simulink model "initial_model2a"  (R2017b)
settings: Solver=ode4  StartTime=0.0  StopTime=time_final  FixedStep=time_step  RelTol=1e-3  AbsTol=1e-6
values from neighbouring files (symbols this model uses):
  A_frontal = 2.8    [tesla_sim_data2.m]    (also in tesla_sim_data2a.m)
  ap00 = -69.58    [tesla_sim_data2.m]    (also in tesla_sim_data2a.m)
  ap01 = 11.22    [tesla_sim_data2.m]    (also in tesla_sim_data2a.m)
  ap02 = -0.1665    [tesla_sim_data2.m]    (also in tesla_sim_data2a.m)
  ap03 = 0.0006218    [tesla_sim_data2.m]    (also in tesla_sim_data2a.m)
  ap10 = 0.5123    [tesla_sim_data2.m]    (also in tesla_sim_data2a.m)
  ap11 = 0.009736    [tesla_sim_data2.m]    (also in tesla_sim_data2a.m)
  ap12 = 0.0003316    [tesla_sim_data2.m]    (also in tesla_sim_data2a.m)
  ap20 = -0.0007943    [tesla_sim_data2.m]    (also in tesla_sim_data2a.m)
  ap21 = -4.587e-07    [tesla_sim_data2.m]    (also in tesla_sim_data2a.m)
  ap30 = 3.794e-07    [tesla_sim_data2.m]    (also in tesla_sim_data2a.m)
  C_d = 0.24    [tesla_sim_data2.m]    (also in tesla_sim_data2a.m)
  enable_stop = 1    [tesla_sim_data2.m]    (also in tesla_sim_data2a.m)
  ess_cap_scale = 1    [tesla_sim_data2.m]    (also in tesla_sim_data2a.m)
  ess_fixtemp = 25    [tesla_sim_data2.m]    (also in tesla_sim_data2a.m)
  ess_max_ah_cap = ess_max_kwhr_cap*1000/350*[1 1]    [tesla_sim_data2.m]    (also in tesla_sim_data2a.m)
  ess_max_volts = 9    [tesla_sim_data2.m]    (also in tesla_sim_data2a.m)
  ess_min_volts = 6    [tesla_sim_data2.m]    (also in tesla_sim_data2a.m)
  ess_module_num = 40    [tesla_sim_data2.m]    (also in tesla_sim_data2a.m)
  ess_r_chg = [ ... (first row only)    [tesla_sim_data2.m]    (also in tesla_sim_data2a.m)
  ess_r_dis = [ ... (first row only)    [tesla_sim_data2.m]    (also in tesla_sim_data2a.m)
  ess_res_scale_coef = [1 0 1 0]    [tesla_sim_data2.m]    (also in tesla_sim_data2a.m)
  ess_res_scale_fun = inline('(x(1)*ess_module_num+x(2))/(x(3)*ess_cap_scale+x(4))','x','ess_module_num','ess_cap_scale')    [tesla_sim_data2.m]    (also in tesla_sim_data2a.m)
  ess_soc = [0 0.1 0.2 0.3 0.4 0.5 0.6 0.7 0.8 0.9 1]    [tesla_sim_data2.m]    (also in tesla_sim_data2a.m)
  ess_tmp = [0 25]    [tesla_sim_data2.m]    (also in tesla_sim_data2a.m)
  ess_voc = [ ... (first row only)    [tesla_sim_data2.m]    (also in tesla_sim_data2a.m)
  f_rolling = 0.018    [tesla_sim_data2.m]    (also in tesla_sim_data2a.m)
  FR = 9.73    [tesla_sim_data2.m]    (also in tesla_sim_data2a.m)
  g_gravity = 9.81    [tesla_sim_data2.m]    (also in tesla_sim_data2a.m)
  m_map_spd = [0	100	250	500	1000	1500	2000	2500	3000	4000	4500	5500	6000	7000	8000	9000	10000]*(2*pi)/60    [tesla_sim_data2.m]    (also in tesla_sim_data2a.m)
  m_max_trq_IM = min(m_peak_trq_IM, m_peak_pwr*1000./m_map_spd)    [tesla_sim_data2.m]    (also in tesla_sim_data2a.m)
  m_max_trq_SR = min(m_peak_trq_SR, m_peak_pwr*1000./m_map_spd)    [tesla_sim_data2.m]    (also in tesla_sim_data2a.m)
  m_min_volts = 200    [tesla_sim_data2.m]    (also in tesla_sim_data2a.m)
  m_peak_pwr = 310    [tesla_sim_data2.m]    (also in tesla_sim_data2a.m)
  M_total = (4650+300)/2.2046    (= 2245.3052708)    [tesla_sim_data2.m]    (also in tesla_sim_data2a.m)
  mtr_speed_rad = linspace(0,6000*2*pi/60,d)    [tesla_sim_data2.m]    (also in tesla_sim_data2a.m = linspace(10,6000*2*pi/60,d))
  mtr_torque_Nm = linspace(0,1000,d)    [tesla_sim_data2.m]    (also in tesla_sim_data2a.m = linspace(10,1600,d))
  p00 = -215.8    [tesla_sim_data2.m]    (also in tesla_sim_data2a.m)
  p01 = 3.368    [tesla_sim_data2.m]    (also in tesla_sim_data2a.m)
  p02 = -0.0178    [tesla_sim_data2.m]    (also in tesla_sim_data2a.m)
  p03 = 6.515e-05    [tesla_sim_data2.m]    (also in tesla_sim_data2a.m)
  p10 = 4.164    [tesla_sim_data2.m]    (also in tesla_sim_data2a.m)
  p11 = 0.04408    [tesla_sim_data2.m]    (also in tesla_sim_data2a.m)
  p12 = 9.874e-05    [tesla_sim_data2.m]    (also in tesla_sim_data2a.m)
  p20 = -0.009417    [tesla_sim_data2.m]    (also in tesla_sim_data2a.m)
  p21 = 5.981e-06    [tesla_sim_data2.m]    (also in tesla_sim_data2a.m)
  p30 = 5.161e-06    [tesla_sim_data2.m]    (also in tesla_sim_data2a.m)
  R_tire = 0.335    [tesla_sim_data2.m]    (also in tesla_sim_data2a.m)
  rho_air = 1.2    [tesla_sim_data2.m]    (also in tesla_sim_data2a.m)
undefined symbols (not defined in the file or in its folder): cyc_mph, ess_init_soc, K_high, K_low, Kp_c, opt_output_torque_location2a, regstop_soc, Ti_c, time_final, Tt_c, v_max_c
libraries: simulink x4
(part 2 of 2)

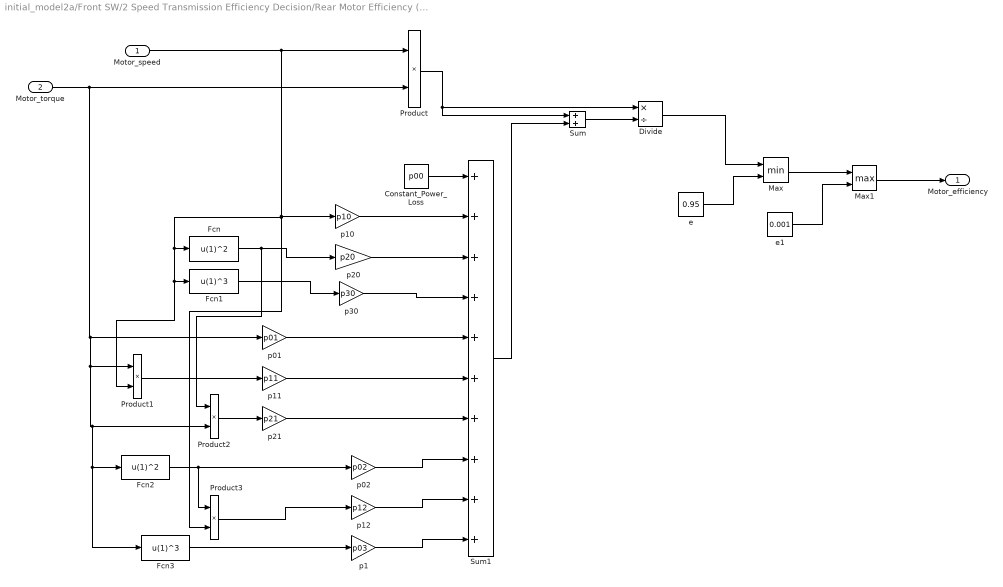
== system initial_model2a/Front SW/2 Speed Transmission Efficiency Decision/Rear Motor Efficiency (K_low) ==
  Motor_speed : Inport
  Motor_torque : Inport  Port=2
  Constant_Power_Loss : Constant  Value=p00
  Divide : Product  Inputs=*/
  Fcn : Fcn  Expr=u(1)^2
  Fcn1 : Fcn  Expr=u(1)^3
  Fcn2 : Fcn  Expr=u(1)^2
  Fcn3 : Fcn  Expr=u(1)^3
  Max : MinMax  Inputs=2
  Max1 : MinMax  Function=max  Inputs=2
  Product{,1..3} (4 alike) : Product
  Sum : Sum
  Sum1 : Sum  Inputs=++++++++++
  e : Constant  Value=0.95
  e1 : Constant  Value=0.001
  p01 : Gain  Gain=p01
  p02 : Gain  Gain=p02
  p1 : Gain  Gain=p03
  p10 : Gain  Gain=p10
  p11 : Gain  Gain=p11
  p12 : Gain  Gain=p12
  p20 : Gain  Gain=p20
  p21 : Gain  Gain=p21
  p30 : Gain  Gain=p30
  Motor_efficiency : Outport
  wires:
  e/1 -> Max/2
  Fcn3/1 -> p1/1
  p1/1 -> Sum1/10
  p12/1 -> Sum1/9
  Product3/1 -> p12/1
  Motor_torque/1 -> Product/2, p01/1, Product1/1, Product2/2, Fcn2/1, Fcn3/1
  p01/1 -> Sum1/5
  p11/1 -> Sum1/6
  p21/1 -> Sum1/7
  p02/1 -> Sum1/8
  Fcn2/1 -> p02/1, Product3/1
  Product2/1 -> p21/1
  Product1/1 -> p11/1
  p30/1 -> Sum1/4
  Fcn1/1 -> p30/1
  Fcn/1 -> p20/1, Product2/1
  p20/1 -> Sum1/3
  p10/1 -> Sum1/2
  Constant_Power_Loss/1 -> Sum1/1
  Motor_speed/1 -> Product/1, p10/1, Fcn/1, Fcn1/1, Product1/2, Product3/2
  Divide/1 -> Max/1
  Sum1/1 -> Sum/2
  Sum/1 -> Divide/2
  Product/1 -> Divide/1, Sum/1
  Max/1 -> Max1/1
  Max1/1 -> Motor_efficiency/1
  e1/1 -> Max1/2

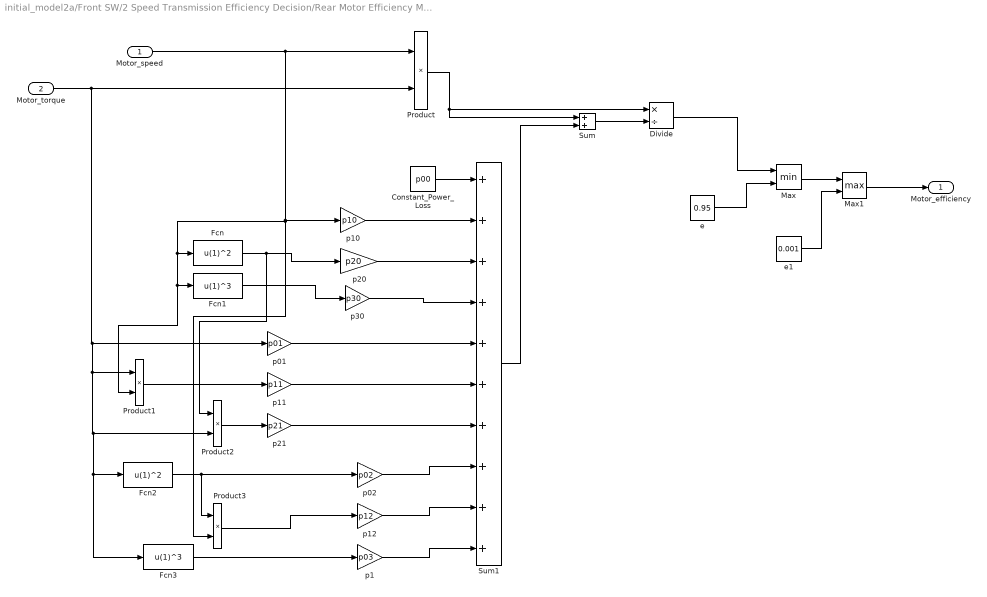
== system initial_model2a/Front SW/2 Speed Transmission Efficiency Decision/Rear Motor Efficiency Map (K_high) ==
  Motor_speed : Inport
  Motor_torque : Inport  Port=2
  Constant_Power_Loss : Constant  Value=p00
  Divide : Product  Inputs=*/
  Fcn : Fcn  Expr=u(1)^2
  Fcn1 : Fcn  Expr=u(1)^3
  Fcn2 : Fcn  Expr=u(1)^2
  Fcn3 : Fcn  Expr=u(1)^3
  Max : MinMax  Inputs=2
  Max1 : MinMax  Function=max  Inputs=2
  Product{,1..3} (4 alike) : Product
  Sum : Sum
  Sum1 : Sum  Inputs=++++++++++
  e : Constant  Value=0.95
  e1 : Constant  Value=0.001
  p01 : Gain  Gain=p01
  p02 : Gain  Gain=p02
  p1 : Gain  Gain=p03
  p10 : Gain  Gain=p10
  p11 : Gain  Gain=p11
  p12 : Gain  Gain=p12
  p20 : Gain  Gain=p20
  p21 : Gain  Gain=p21
  p30 : Gain  Gain=p30
  Motor_efficiency : Outport
  wires:
  e/1 -> Max/2
  Fcn3/1 -> p1/1
  p1/1 -> Sum1/10
  p12/1 -> Sum1/9
  Product3/1 -> p12/1
  Motor_torque/1 -> Product/2, p01/1, Product1/1, Product2/2, Fcn2/1, Fcn3/1
  p01/1 -> Sum1/5
  p11/1 -> Sum1/6
  p21/1 -> Sum1/7
  p02/1 -> Sum1/8
  Fcn2/1 -> p02/1, Product3/1
  Product2/1 -> p21/1
  Product1/1 -> p11/1
  p30/1 -> Sum1/4
  Fcn1/1 -> p30/1
  Fcn/1 -> p20/1, Product2/1
  p20/1 -> Sum1/3
  p10/1 -> Sum1/2
  Constant_Power_Loss/1 -> Sum1/1
  Motor_speed/1 -> Product/1, p10/1, Fcn/1, Fcn1/1, Product1/2, Product3/2
  Divide/1 -> Max/1
  Sum1/1 -> Sum/2
  Sum/1 -> Divide/2
  Product/1 -> Divide/1, Sum/1
  Max/1 -> Max1/1
  Max1/1 -> Motor_efficiency/1
  e1/1 -> Max1/2

== system initial_model2a/Hybrid Controller/Brake/Regen Control ==
  soc : Inport
  veh sped : Inport  Port=2
  Logical Operator : Logic  Inputs=3
  regen swith on : Constant
  soc < soc_stopcharging : Relay  OnSwitchValue=regstop_soc  OffSwitchValue=regstop_soc  OnOutputValue=0  OffOutputValue=1
  veh spd>= 0.4 mph : Relay  OnSwitchValue=0.4  OffSwitchValue=0.4
  "Use regen? " : Outport
  wires:
  veh sped/1 -> veh spd>= 0.4 mph/1
  soc/1 -> soc < soc_stopcharging/1
  veh spd>= 0.4 mph/1 -> Logical Operator/1
  Logical Operator/1 -> "Use regen? "/1
  soc < soc_stopcharging/1 -> Logical Operator/2
  regen swith on/1 -> Logical Operator/3
